simulink model "Controlled_DoubleTank_real"  (R2014a)
settings: Solver=ode1  StartTime=0.0  StopTime=inf  FixedStep=0.02  RelTol=1e-3
PostLoadFcn:
  | qc_set_target_type(getConfigSet(bdroot, 'QUARC Default Target Configuration'));
values from neighbouring files (symbols this model uses):
  A = [0.967743748526  0; 0.031730333008  0.967743748526]    [Dados_Tanques.mat]    (also in double_tank_simu.m = sysd.A; nma_simplex.m = tab(1:nRow-1,1:nCol-1); nma_simplex_2.m = tab(1:nRow-1,1:nCol-1))
  B = [0.104604453049 0.0017055116738]    [Dados_Tanques.mat]    (also in double_tank_simu.m = sysd.B)
  Gv = [1 -1 0 0 0.0316763086938 -0.0316763086938 0.0610064360648 -0.0610064360648 0.0878578258116 -0.0878578258116 0.112163466595 -0.112163466595 ... (32 elements, 16x2)]    [Dados_Tanques.mat]
  phi = [2.74907887757 9.25092112243]    [Dados_Tanques.mat]    (also in double_tank_simu.m = [(12-ueq) ueq]')
  rhov = [15 15 15 15 14.8404669643 14.8293968766 14.6652011254 14.6221983313 14.4769073428 14.3832726141 14.2782768412 14.1176408708 ... (16 elements, 16x1)]    [Dados_Tanques.mat]
  U = [1 -1]    [Dados_Tanques.mat]    (also in double_tank_simu.m = [1 -1]')
  ueq = 9.25092112243    [Dados_Tanques.mat]    (also in double_tank_simu.m = (a1/km)*sqrt(2*g*x1eq))
  x1eq = 15    [Dados_Tanques.mat]    (also in double_tank_simu.m = (1/(2*g))*((km*ueq)/a1)^2)
  x2eq = 15    [Dados_Tanques.mat]    (also in double_tank_simu.m)
undefined symbols (not defined in the file or in its folder): HIL
libraries: quarc_library x3
settings Model: SimulationMode=external  ExtModeTrigDuration=30000  Creator=MLevis  LastModifiedBy=aluno
settings SolverCC: PositivePriorityOrder=on
settings DataIOCC: SignalLoggingSaveFormat=ModelDataLogs
settings OptimizationCC: ExpressionDepthLimit=2147483647  InitFltsAndDblsToZero=on
settings DebuggingCC: SaveWithParameterizedLinksMsg=none  UnderspecifiedInitializationDetection=Classic  MultiTaskDSMMsg=warning  MultiTaskCondExecSysMsg=none  FcnCallInpInsideContextMsg=UseLocalSettings  StateNameClashWarn=warning
settings RTWCC: SystemTargetFile=quarc_win64.tlc  TemplateMakefile=quarc_default_tmf  Description=QUARC Win64 Target  ProcessScript=quarc_win64_make_rtw_hook
settings STFCustomTargetCC: CPPClassGenCompliant=on
settings GRTTargetCC: ParMdlRefBuildCompliant=off  CompOptLevelCompliant=off  CombineOutputUpdateFcns=off  MatFileLogging=off  GRTInterface=on  ExtMode=on  ExtModeMexFile=quarc_comm

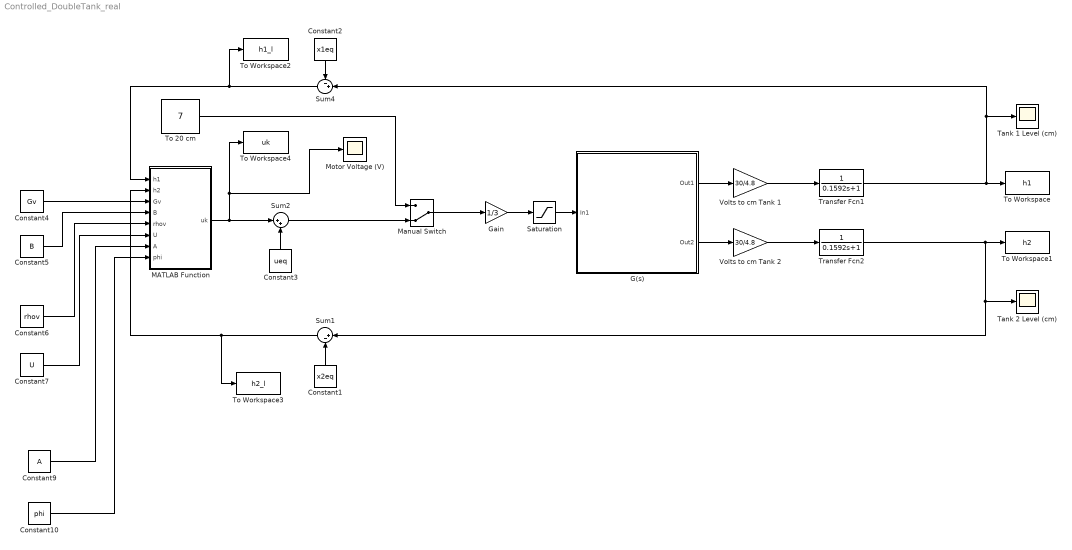
== system Controlled_DoubleTank_real ==
  Constant1 : Constant  Value=x2eq
  Constant10 : Constant  Value=phi
  Constant2 : Constant  Value=x1eq
  Constant3 : Constant  Value=ueq
  Constant4 : Constant  Value=Gv
  Constant5 : Constant  Value=B
  Constant6 : Constant  Value=rhov
  Constant7 : Constant  Value=U
  Constant9 : Constant  Value=A
  G(s) : Subsystem
  Gain : Gain  Gain=1/3
  MATLAB Function : MATLAB Function  TreatAsAtomicUnit=on
  Manual Switch : ManualSwitch  CurrentSetting=0
  Motor Voltage (V) : Scope
      settings: TimeRange=30  YMin=5.5  YMax=12
  Saturation : Saturate  UpperLimit=4  LowerLimit=-4
  Sum1 : Sum  Inputs=|+-
  Sum2 : Sum  Inputs=|++
  Sum4 : Sum  Inputs=-+|
  Tank 1 Level (cm) : Scope
      settings: TimeRange=100  YMin=-2.5  YMax=30  SaveName=ScopeData2
  Tank 2 Level (cm) : Scope
      settings: TimeRange=100  YMin=0  YMax=30
  To 20 cm : Constant  Value=7
  To Workspace : ToWorkspace  VariableName=h1  SaveFormat=Timeseries  SampleTime=-1
  To Workspace1 : ToWorkspace  VariableName=h2  SaveFormat=Timeseries  SampleTime=-1
  To Workspace2 : ToWorkspace  VariableName=h1_l  SaveFormat=Timeseries  SampleTime=-1
  To Workspace3 : ToWorkspace  VariableName=h2_l  SaveFormat=Timeseries  SampleTime=-1
  To Workspace4 : ToWorkspace  VariableName=uk  SaveFormat=Timeseries  SampleTime=-1
  Transfer Fcn1 : TransferFcn  Denominator=[0.1592 1]
  Transfer Fcn2 : TransferFcn  Denominator=[0.1592 1]
  Volts to cm Tank 1 : Gain  Gain=30/4.8
  Volts to cm Tank 2 : Gain  Gain=30/4.8
  wires:
  Transfer Fcn1/1 -> Tank 1 Level (cm)/1, Sum4/2, To Workspace/1
  Transfer Fcn2/1 -> Sum1/1, Tank 2 Level (cm)/1, To Workspace1/1
  Sum4/1 -> MATLAB Function/1(h1), To Workspace2/1
  Constant2/1 -> Sum4/1
  Constant1/1 -> Sum1/2
  Sum1/1 -> MATLAB Function/2(h2), To Workspace3/1
  Constant3/1 -> Sum2/2
  Sum2/1 -> Manual Switch/2
  MATLAB Function/1(uk) -> Sum2/1, Motor Voltage (V)/1, To Workspace4/1
  Gain/1 -> Saturation/1
  G(s)/1(Out1) -> Volts to cm Tank 1/1
  Volts to cm Tank 2/1 -> Transfer Fcn2/1
  G(s)/2(Out2) -> Volts to cm Tank 2/1
  Volts to cm Tank 1/1 -> Transfer Fcn1/1
  Saturation/1 -> G(s)/1(In1)
  To 20 cm/1 -> Manual Switch/1
  Manual Switch/1 -> Gain/1
  Constant4/1 -> MATLAB Function/3(Gv)
  Constant5/1 -> MATLAB Function/4(B)
  Constant6/1 -> MATLAB Function/5(rhov)
  Constant7/1 -> MATLAB Function/6(U)
  Constant9/1 -> MATLAB Function/7(A)
  Constant10/1 -> MATLAB Function/8(phi)

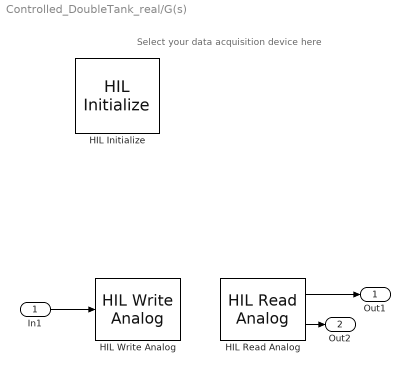
== system Controlled_DoubleTank_real/G(s) ==
  note: Select your data acquisition device here
  In1 : Inport
  HIL Initialize : quarc_library/Data Acquisition/Generic/Configuration/HIL Initialize  object_name=HIL-1  board_type=q2_usb  board_number=0  board_options=d0=digital;d1=digital;led=auto;update_rate=normal;decimation=1  exclusive=off  active=off  hardware_clocks=[0]  clock_modes=[]  initial_clock_frequencies=[]  set_clock_params_at_start=off  set_clock_params_at_switch_in=off  set_clock_frequencies_at_start=off  set_clock_frequencies_at_switch_in=off  analog_input_channels=[0:1]  analog_input_maximums=10  analog_input_minimums=-10  set_analog_input_params_at_start=on  set_analog_input_params_at_switch_in=off  analog_output_channels=[0:1]  analog_output_maximums=10  analog_output_minimums=-10  initial_analog_outputs=[0]  final_analog_outputs=[0]  watchdog_analog_outputs=0  set_analog_output_params_at_start=on  set_analog_output_params_at_switch_in=off  set_analog_outputs_at_start=on  set_analog_outputs_at_switch_in=off  set_analog_outputs_at_terminate=on  set_analog_outputs_at_switch_out=off  set_analog_outputs_on_watchdog=off  digital_input_channels=[]  digital_output_channels=[]  digital_output_configuration=[]  initial_digital_outputs=[1]  final_digital_outputs=[1]  watchdog_digital_outputs=[1]  set_digital_output_params_at_start=off  set_digital_output_params_at_switch_in=off  set_digital_outputs_at_start=on  set_digital_outputs_at_switch_in=off  set_digital_outputs_at_terminate=on  set_digital_outputs_at_switch_out=off  set_digital_outputs_on_watchdog=off  encoder_channels=[0:1]  quadrature=[4]  encoder_filter_frequency=[]  initial_encoder_counts=[0]  set_encoder_params_at_start=on  set_encoder_params_at_switch_in=off  set_encoder_counts_at_start=on  set_encoder_counts_at_switch_in=off  pwm_channels=[]  pwm_modes=[0]  pwm_frequency=1/0.020  pwm_configuration=[]  pwm_alignment=[]  pwm_polarity=[]  pwm_leading_deadband=[]  pwm_trailing_deadband=[]  initial_pwm_outputs=[0]  final_pwm_outputs=[0]  watchdog_pwm_outputs=[0]  set_pwm_params_at_start=on  set_pwm_params_at_switch_in=off  set_pwm_outputs_at_start=on  set_pwm_outputs_at_switch_in=off  set_pwm_outputs_at_terminate=on  set_pwm_outputs_at_switch_out=off  set_pwm_outputs_on_watchdog=off  other_output_channels=[]  initial_other_outputs=[]  final_other_outputs=[]  watchdog_other_outputs=[]  set_other_outputs_at_start=off  set_other_outputs_at_switch_in=off  set_other_outputs_at_terminate=off  set_other_outputs_at_switch_out=off  set_other_outputs_on_watchdog=off
  HIL Read Analog : quarc_library/Data Acquisition/Generic/Immediate I//O/HIL Read Analog  object_name=HIL-1  channels=[0:1]  sample_time=qc_get_step_size  active=on  vector_output=off
  HIL Write Analog : quarc_library/Data Acquisition/Generic/Immediate I//O/HIL Write Analog  object_name=HIL-1  channels=0  sample_time=-1  active=off  vector_input=off
  Out1 : Outport
  Out2 : Outport  Port=2
  wires:
  HIL Read Analog/1 -> Out1/1
  In1/1 -> HIL Write Analog/1
  HIL Read Analog/2 -> Out2/1

== matlab function Controlled_DoubleTank_real/MATLAB Function ==
  data: h1 input; uk output; h2 input; Gv input; B input; rhov input; U input; A input; phi input
%%%%%%%%%%%%%%%%%%%%%%%%%%%%%%%%%%%%
% STATIC STATE FEEDBACK CONTROLLER %
%%%%%%%%%%%%%%%%%%%%%%%%%%%%%%%%%%%%

function uk = fcn(h1, h2, Gv, B, rhov, U, A, phi)
    % hard-coded paramenters
    ncu = 1;
    nlu = 2;
    
    %coder.extrinsic('nma_simplex');
    xk = [h1 h2]';
    c = [zeros(ncu, 1) 1 zeros(1,18)];
    Aa = [[Gv*B -rhov; U zeros(nlu, 1)] eye(18)];
    b = [-Gv*A*xk; phi];

    %====== NMA_SIMPLEX
    %===== validate_input(Aa,b,c);
    if ~ismatrix(Aa)
        error('A must be matrix');
    end
    
    if ~isvector(b)
        error('b must be vector');
    end
    if ~isvector(c)
        error('c must be vector');
    end
    
    [m,n]=size(Aa);
    if rank(Aa) <m
        error('Rank A must be equal to number of rows in A');
    end
    
    if length(b) ~= m
        error('b must have same size as number of rows of A');
    end
    if length(c) ~= n
        error('c must have same size as number of columns of A');
    end
    %===== end validate_input(Aa,b,c);

    %==== [Aa,b] = make_phase_one(Aa,b,debug);
    [m_aux,n_aux]              = size(Aa);
    tab                = zeros(m_aux+1,n_aux+m_aux+1);
    tab(1:m_aux,1:n_aux)       = Aa;
    tab(end,n_aux+1:end-1) = 1;
    tab(1:m_aux,end)       = b(:);
    tab(1:m_aux,n_aux+1:n_aux+m_aux)   = eye(m_aux);

    for i = 1:m_aux %now make all entries in bottom row zero
        tab(end,:) = tab(end,:)-tab(i,:);
    end

    %==== tab = simplex(tab(1:m,1:n+m),tab(1:m,end),tab(end,1:n+m),debug,'phase one');
    Aa_aux = tab(1:m,1:n+m)
    b_aux = tab(1:m,end)
    c_aux = tab(end,1:n+m)

    [m,n]        = size(Aa_aux);
    tab          = zeros(m+1,n+1);
    tab(1:m,1:n) = Aa_aux;
    tab(m+1,1:n) = c_aux(:);
    tab(1:m,end) = b_aux(:);

    keep_running = true;
    while keep_running
        
        if any(tab(end,1:n)<0)%check if there is negative cost coeff.
            [~,J] = min(tab(end,1:n)); %yes, find the most negative
            % now check if corresponding column is unbounded
            if all(tab(1:m,J)<=0) 
            error('problem unbounded. All entries <= 0 in column %d',J);
            %do row operations to make all entries in the column 0 
            %except pivot
            else 
                pivot_row = 0;
                min_found = inf;
                for i = 1:m
                    if tab(i,J)>0
                        tmp = tab(i,end)/tab(i,J);
                        if tmp < min_found
                            min_found = tmp;
                            pivot_row = i;
                        end
                    end
                end
                %normalize
                tab(pivot_row,:) = tab(pivot_row,:)/tab(pivot_row,J); 
                %now make all entries in J column zero.
                for i=1:m+1
                    if i ~= pivot_row
                        tab(i,:)=tab(i,:)-sign(tab(i,J))*...
                                    abs(tab(i,J))*tab(pivot_row,:);
                    end
                end
            end
        else
            keep_running=false;       
        end
    end
    %==== END tab = simplex(tab(1:m,1:n+m),tab(1:m,end),tab(end,1:n+m),debug,'phase one');

    Aa = tab(1:m_aux,1:n_aux);
    b = tab(1:m_aux,end);
    %==== end [Aa,b] = make_phase_one(Aa,b,debug);

    %==== tab = simplex(Aa,b,c,debug,'phase two')
    [m,n]        = size(Aa);
    tab          = zeros(m+1,n+1);
    tab(1:m,1:n) = Aa;
    tab(m+1,1:n) = c(:);
    tab(1:m,end) = b(:);

    keep_running = true;
    while keep_running
        
        if any(tab(end,1:n)<0)%check if there is negative cost coeff.
            [~,J] = min(tab(end,1:n)); %yes, find the most negative
            % now check if corresponding column is unbounded
            if all(tab(1:m,J)<=0) 
            error('problem unbounded. All entries <= 0 in column %d',J);
            %do row operations to make all entries in the column 0 
            %except pivot
            else 
                pivot_row = 0;
                min_found = inf;
                for i = 1:m
                    if tab(i,J)>0
                        tmp = tab(i,end)/tab(i,J);
                        if tmp < min_found
                            min_found = tmp;
                            pivot_row = i;
                        end
                    end
                end
                %normalize
                tab(pivot_row,:) = tab(pivot_row,:)/tab(pivot_row,J); 
                %now make all entries in J column zero.
                for i=1:m+1
                    if i ~= pivot_row
                        tab(i,:)=tab(i,:)-sign(tab(i,J))*...
                                    abs(tab(i,J))*tab(pivot_row,:);
                    end
                end
            end
        else
            keep_running=false;       
        end
    end
    %==== END tab = simplex(Aa,b,c,debug,'phase two')
    
    %==== sol = print_solution_vector(tab);
    [nRow,nCol] = size(tab);

    A = tab(1:nRow-1,1:nCol-1);
    b = tab(1:nRow-1,nCol);

    q = A ~= 0;
    q = find(sum(q,1)==1); %find all columns with one non-zero entry;

    sol = zeros(nCol-1,1); 

    for n=1:length(q)
        j = find(A(1:nRow-1,q(n))==1);
        if isempty(j)
        sol(q(n)) = 0;
        else
        sol(q(n)) = b(j); 
        end
    end
    %==== END sol = print_solution_vector(tab);
    %====== END NMA_SIMPLEX
    
    uk = sol(1);
end
